simulink model "platoon_plus"  (R2020b)
settings: Solver=VariableStepAuto  StartTime=0.0  StopTime=120  RelTol=1e-3
values from neighbouring files (symbols this model uses):
  d_0 = 8    [platoon.m]
  Ka = 0.55    [platoon.m]
  Kd_err_pl = 0.401    [platoon.m]
  Kv = 0.5    [platoon.m]
  Kv_r_pl = 0.56    [platoon.m]
  t_h_tar = 1    [platoon.m]
  v_initial = [30 25 28 27]    [platoon.m]
  v_tar = 30    [platoon.m]
  x_initial = [150 100 50 0]    [platoon.m]
libraries: simulink x8
settings Model: Creator=alessandro  LastModifiedBy=gabriele

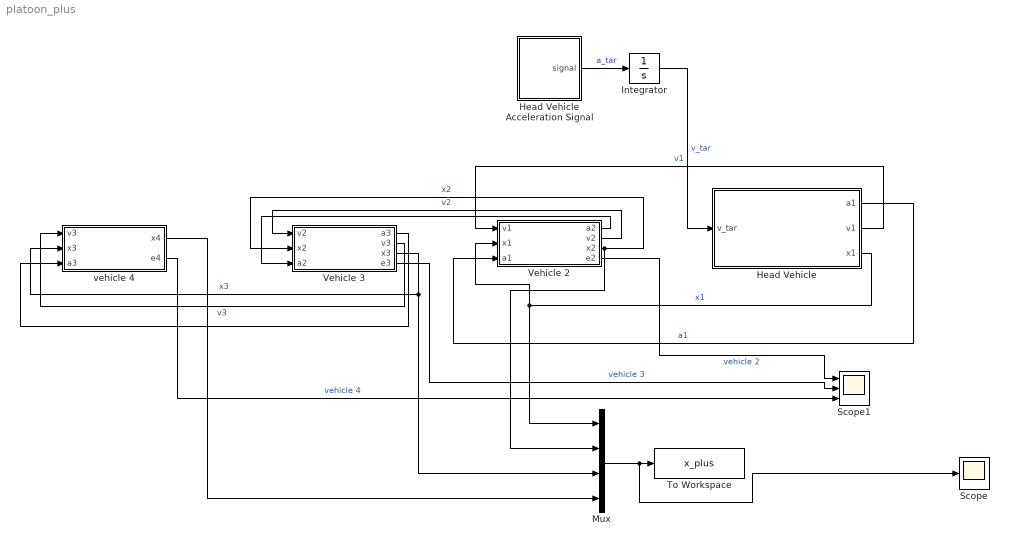
== system platoon_plus ==
  "Head Vehicle " : Subsystem
  Head Vehicle Acceleration Signal : Subsystem
  Integrator : Integrator  InitialCondition=v_initial(1)
  Mux : Mux
  Scope : Scope
  Scope1 : Scope  NumInputPorts=3
  To Workspace : ToWorkspace  VariableName=x_plus  SampleTime=-1
  Vehicle 2 : Subsystem
  Vehicle 3 : Subsystem
  vehicle 4 : Subsystem
  wires:
  Mux/1 -> Scope/1, To Workspace/1
  Vehicle 2/2(v2) -> Vehicle 3/1(v2)  "v2"
  Head Vehicle Acceleration Signal/1(signal) -> Integrator/1  "a_tar"
  vehicle 4/1(x4) -> Mux/4
  "Head Vehicle "/2(v1) -> Vehicle 2/1(v1)  "v1"
  Vehicle 3/2(v3) -> vehicle 4/1(v3)  "v3"
  Integrator/1 -> "Head Vehicle "/1(v_tar)  "v_tar"
  Vehicle 2/3(x2) -> Mux/2, Vehicle 3/2(x2)  "x2"
  "Head Vehicle "/3(x1) -> Mux/1, Vehicle 2/2(x1)  "x1"
  Vehicle 3/3(x3) -> Mux/3, vehicle 4/2(x3)  "x3"
  "Head Vehicle "/1(a1) -> Vehicle 2/3(a1)  "a1"
  Vehicle 2/1(a2) -> Vehicle 3/3(a2)
  Vehicle 3/1(a3) -> vehicle 4/3(a3)
  Vehicle 2/4(e2) -> Scope1/1  "vehicle 2"
  Vehicle 3/4(e3) -> Scope1/2  "vehicle 3"
  vehicle 4/2(e4) -> Scope1/3  "vehicle 4"

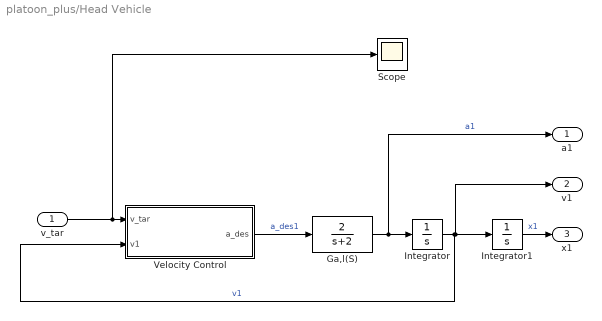
== system platoon_plus/Head Vehicle  ==
  v_tar : Inport
  Ga,l(S) : TransferFcn  Numerator=[2]  Denominator=[1 2]
  Integrator : Integrator  InitialCondition=v_initial(1)
  Integrator1 : Integrator  InitialCondition=x_initial(1)
  Scope : Scope
  Velocity Control : Subsystem
  a1 : Outport
  v1 : Outport  Port=2
  x1 : Outport  Port=3
  wires:
  Integrator/1 -> Velocity Control/2(v1), v1/1, Integrator1/1  "v1"
  Ga,l(S)/1 -> a1/1, Integrator/1  "a1"
  v_tar/1 -> Scope/1, Velocity Control/1(v_tar)
  Velocity Control/1(a_des) -> Ga,l(S)/1  "a_des1"
  Integrator1/1 -> x1/1  "x1"

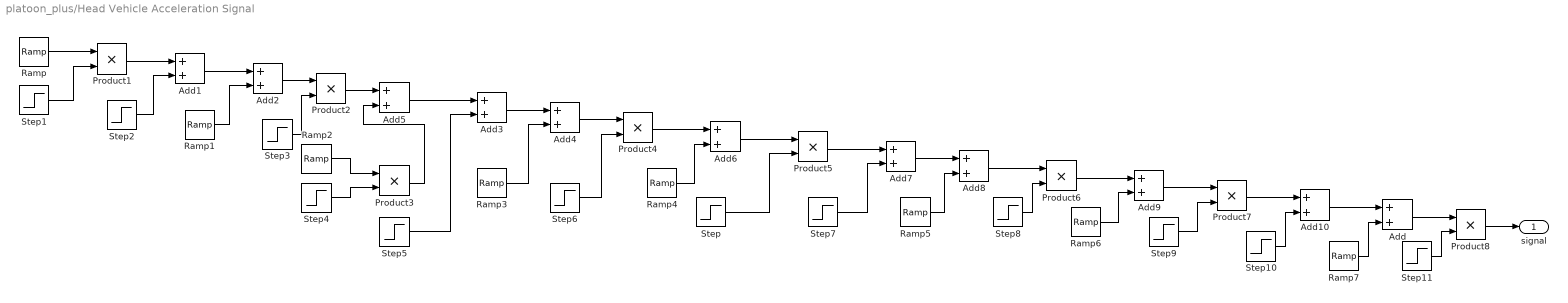
== system platoon_plus/Head Vehicle Acceleration Signal ==
  Add{,1..10} (11 alike) : Sum
  Product{1..8} (8 alike) : Product
  Ramp : simulink/Sources/Ramp  slope=-4  start=10  InitialOutput=0
  Ramp1 : simulink/Sources/Ramp  slope=4  start=13.5  InitialOutput=0
  Ramp2 : simulink/Sources/Ramp  slope=4  start=40  InitialOutput=0
  Ramp3 : simulink/Sources/Ramp  slope=-4  start=43.5  InitialOutput=0
  Ramp4 : simulink/Sources/Ramp  slope=-4  start=70  InitialOutput=0
  Ramp5 : simulink/Sources/Ramp  slope=4  start=73.5  InitialOutput=0
  Ramp6 : simulink/Sources/Ramp  slope=4  start=100  InitialOutput=0
  Ramp7 : simulink/Sources/Ramp  slope=-4  start=103.5  InitialOutput=0
  Step : Step  Time=70.5  Before=1  After=0  SampleTime=0
  Step1 : Step  Time=10.5  Before=1  After=0  SampleTime=0.1
  Step10 : Step  Time=100.5  After=2  SampleTime=0
  Step11 : Step  Time=104  Before=1  After=0  SampleTime=0
  Step2 : Step  Time=10.5  After=-2  SampleTime=0
  Step3 : Step  Time=14  Before=1  After=0  SampleTime=0
  Step4 : Step  Time=40.5  Before=1  After=0  SampleTime=0
  Step5 : Step  Time=40.5  After=2  SampleTime=0
  Step6 : Step  Time=44  Before=1  After=0  SampleTime=0
  Step7 : Step  Time=70.5  After=-2  SampleTime=0
  Step8 : Step  Time=74  Before=1  After=0  SampleTime=0
  Step9 : Step  Time=100.5  Before=1  After=0  SampleTime=0
  signal : Outport
  wires:
  Add1/1 -> Add2/1
  Step3/1 -> Product2/2
  Product3/1 -> Add5/2
  Step5/1 -> Add3/2
  Add2/1 -> Product2/1
  Step1/1 -> Product1/2
  Product2/1 -> Add5/1
  Step2/1 -> Add1/2
  Ramp2/1 -> Product3/1
  Product1/1 -> Add1/1
  Add4/1 -> Product4/1
  Ramp/1 -> Product1/1
  Add3/1 -> Add4/1
  Step6/1 -> Product4/2
  Ramp1/1 -> Add2/2
  Step4/1 -> Product3/2
  Add5/1 -> Add3/1
  Ramp3/1 -> Add4/2
  Product4/1 -> Add6/1
  Ramp4/1 -> Add6/2
  Add6/1 -> Product5/1
  Step/1 -> Product5/2
  Product5/1 -> Add7/1
  Step7/1 -> Add7/2
  Add7/1 -> Add8/1
  Ramp5/1 -> Add8/2
  Add8/1 -> Product6/1
  Step8/1 -> Product6/2
  Product6/1 -> Add9/1
  Ramp6/1 -> Add9/2
  Add9/1 -> Product7/1
  Step9/1 -> Product7/2
  Step10/1 -> Add10/2
  Product7/1 -> Add10/1
  Add10/1 -> Add/1
  Ramp7/1 -> Add/2
  Add/1 -> Product8/1
  Step11/1 -> Product8/2
  Product8/1 -> signal/1

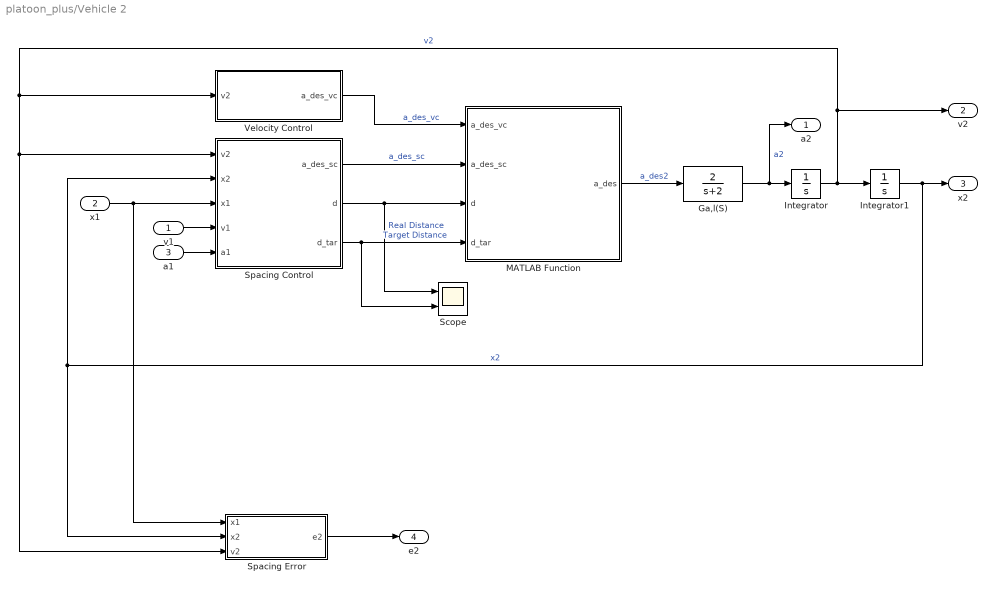
== system platoon_plus/Vehicle 2 ==
  v1 : Inport
  x1 : Inport  Port=2
  a1 : Inport  Port=3
  Ga,l(S) : TransferFcn  Numerator=[2]  Denominator=[1 2]
  Integrator : Integrator  InitialCondition=v_initial(2)
  Integrator1 : Integrator  InitialCondition=x_initial(2)
  MATLAB Function : MATLAB Function  TreatAsAtomicUnit=on
  Scope : Scope  NumInputPorts=2
  Spacing Control : Subsystem
  Spacing Error : Subsystem
  Velocity Control : Subsystem
  a2 : Outport
  v2 : Outport  Port=2
  x2 : Outport  Port=3
  e2 : Outport  Port=4
  wires:
  Spacing Control/1(a_des_sc) -> MATLAB Function/2(a_des_sc)  "a_des_sc"
  Velocity Control/1(a_des_vc) -> MATLAB Function/1(a_des_vc)  "a_des_vc"
  v1/1 -> Spacing Control/4(v1)
  x1/1 -> Spacing Control/3(x1), Spacing Error/1(x1)
  Spacing Control/2(d) -> Scope/1, MATLAB Function/3(d)  "Real Distance"
  MATLAB Function/1(a_des) -> Ga,l(S)/1  "a_des2"
  Integrator1/1 -> x2/1, Spacing Control/2(x2), Spacing Error/2(x2)  "x2"
  Spacing Control/3(d_tar) -> Scope/2, MATLAB Function/4(d_tar)  "Target Distance"
  Ga,l(S)/1 -> a2/1, Integrator/1  "a2"
  Integrator/1 -> Integrator1/1, v2/1, Velocity Control/1(v2), Spacing Control/1(v2), Spacing Error/3(v2)  "v2"
  Spacing Error/1(e2) -> e2/1
  a1/1 -> Spacing Control/5(a1)

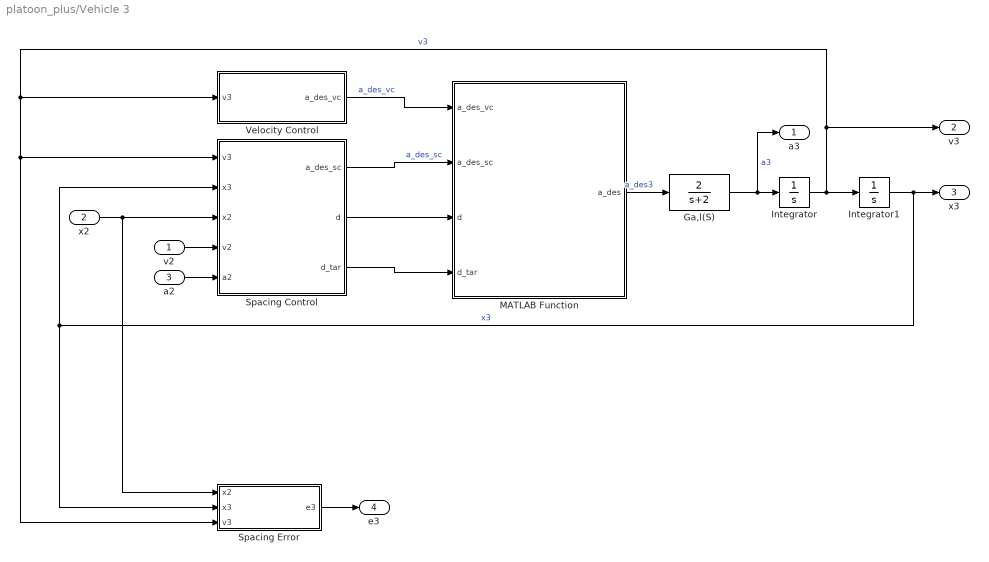
== system platoon_plus/Vehicle 3 ==
  v2 : Inport
  x2 : Inport  Port=2
  a2 : Inport  Port=3
  Ga,l(S) : TransferFcn  Numerator=[2]  Denominator=[1 2]
  Integrator : Integrator  InitialCondition=v_initial(3)
  Integrator1 : Integrator  InitialCondition=x_initial(3)
  MATLAB Function : MATLAB Function  TreatAsAtomicUnit=on
  Spacing Control : Subsystem
  Spacing Error : Subsystem
  Velocity Control : Subsystem
  a3 : Outport
  v3 : Outport  Port=2
  x3 : Outport  Port=3
  e3 : Outport  Port=4
  wires:
  Spacing Control/1(a_des_sc) -> MATLAB Function/2(a_des_sc)  "a_des_sc"
  Velocity Control/1(a_des_vc) -> MATLAB Function/1(a_des_vc)  "a_des_vc"
  v2/1 -> Spacing Control/4(v2)
  x2/1 -> Spacing Control/3(x2), Spacing Error/1(x2)
  Spacing Control/2(d) -> MATLAB Function/3(d)
  MATLAB Function/1(a_des) -> Ga,l(S)/1  "a_des3"
  Integrator1/1 -> x3/1, Spacing Control/2(x3), Spacing Error/2(x3)  "x3"
  Spacing Control/3(d_tar) -> MATLAB Function/4(d_tar)
  Ga,l(S)/1 -> a3/1, Integrator/1  "a3"
  Integrator/1 -> Integrator1/1, v3/1, Velocity Control/1(v3), Spacing Error/3(v3), Spacing Control/1(v3)  "v3"
  Spacing Error/1(e3) -> e3/1
  a2/1 -> Spacing Control/5(a2)

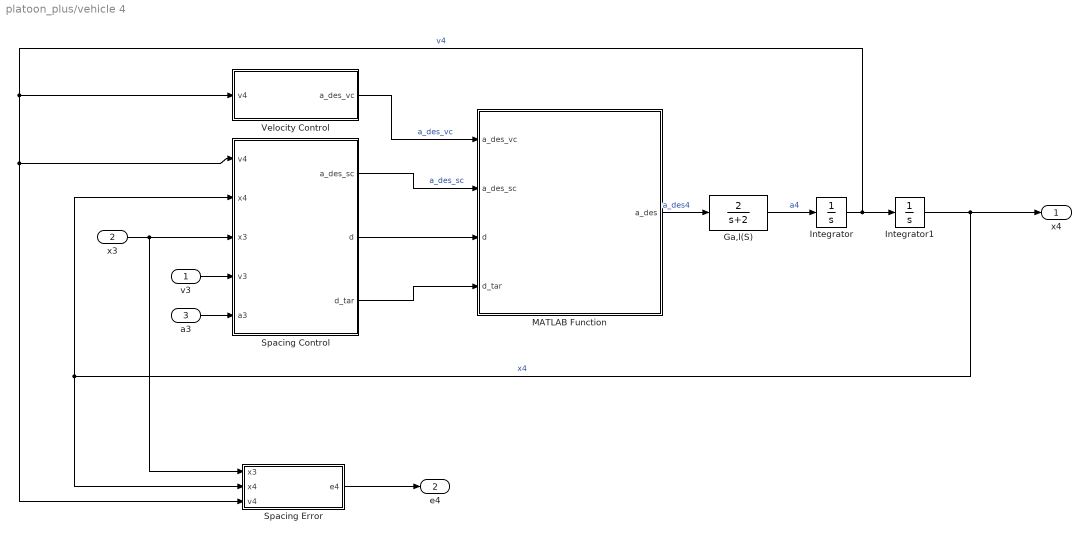
== system platoon_plus/vehicle 4 ==
  v3 : Inport
  x3 : Inport  Port=2
  a3 : Inport  Port=3
  Ga,l(S) : TransferFcn  Numerator=[2]  Denominator=[1 2]
  Integrator : Integrator  InitialCondition=v_initial(4)
  Integrator1 : Integrator  InitialCondition=x_initial(4)
  MATLAB Function : MATLAB Function  TreatAsAtomicUnit=on
  Spacing Control : Subsystem
  Spacing Error : Subsystem
  Velocity Control : Subsystem
  x4 : Outport
  e4 : Outport  Port=2
  wires:
  Spacing Control/1(a_des_sc) -> MATLAB Function/2(a_des_sc)  "a_des_sc"
  Velocity Control/1(a_des_vc) -> MATLAB Function/1(a_des_vc)  "a_des_vc"
  v3/1 -> Spacing Control/4(v3)
  x3/1 -> Spacing Error/1(x3), Spacing Control/3(x3)
  Spacing Control/2(d) -> MATLAB Function/3(d)
  MATLAB Function/1(a_des) -> Ga,l(S)/1  "a_des4"
  Integrator1/1 -> Spacing Control/2(x4), Spacing Error/2(x4), x4/1  "x4"
  Spacing Control/3(d_tar) -> MATLAB Function/4(d_tar)
  Ga,l(S)/1 -> Integrator/1  "a4"
  Integrator/1 -> Integrator1/1, Velocity Control/1(v4), Spacing Error/3(v4), Spacing Control/1(v4)  "v4"
  Spacing Error/1(e4) -> e4/1
  a3/1 -> Spacing Control/5(a3)

== system platoon_plus/Head Vehicle /Velocity Control ==
  v_tar : Inport
  v1 : Inport  Port=2
  Gain : Gain  Gain=Kv
  Subtract : Sum  Inputs=+-
  a_des : Outport
  wires:
  v1/1 -> Subtract/2
  v_tar/1 -> Subtract/1
  Subtract/1 -> Gain/1  "e_v"
  Gain/1 -> a_des/1  "a_des"

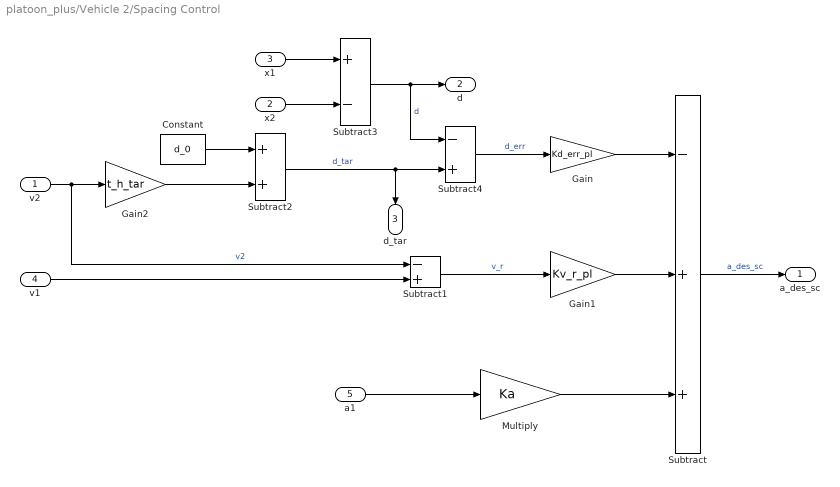
== system platoon_plus/Vehicle 2/Spacing Control ==
  v2 : Inport
  x2 : Inport  Port=2
  x1 : Inport  Port=3
  v1 : Inport  Port=4
  a1 : Inport  Port=5
  Constant : Constant  Value=d_0
  Gain : Gain  Gain=Kd_err_pl
  Gain1 : Gain  Gain=Kv_r_pl
  Gain2 : Gain  Gain=t_h_tar
  Multiply : Gain  Gain=Ka
  Subtract : Sum  Inputs=-++
  Subtract1 : Sum  Inputs=-+
  Subtract2 : Sum
  Subtract3 : Sum  Inputs=+-
  Subtract4 : Sum  Inputs=-+
  a_des_sc : Outport
  d : Outport  Port=2
  d_tar : Outport  Port=3
  wires:
  Gain/1 -> Subtract/1
  Gain1/1 -> Subtract/2
  Subtract/1 -> a_des_sc/1  "a_des_sc"
  v2/1 -> Subtract1/1, Gain2/1  "v2"
  Subtract1/1 -> Gain1/1  "v_r"
  Gain2/1 -> Subtract2/2
  v1/1 -> Subtract1/2
  x1/1 -> Subtract3/1
  x2/1 -> Subtract3/2
  Subtract2/1 -> Subtract4/2, d_tar/1  "d_tar"
  Subtract3/1 -> Subtract4/1, d/1  "d"
  Subtract4/1 -> Gain/1  "d_err"
  Constant/1 -> Subtract2/1
  a1/1 -> Multiply/1
  Multiply/1 -> Subtract/3

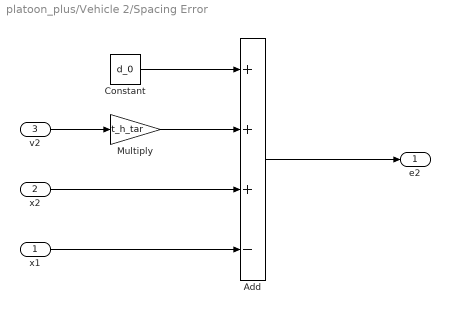
== system platoon_plus/Vehicle 2/Spacing Error ==
  x1 : Inport
  x2 : Inport  Port=2
  v2 : Inport  Port=3
  Add : Sum  Inputs=+++-
  Constant : Constant  Value=d_0
  Multiply : Gain  Gain=t_h_tar
  e2 : Outport
  wires:
  Constant/1 -> Add/1
  Multiply/1 -> Add/2
  v2/1 -> Multiply/1
  x2/1 -> Add/3
  x1/1 -> Add/4
  Add/1 -> e2/1

== system platoon_plus/Vehicle 2/Velocity Control ==
  v2 : Inport
  Constant : Constant  Value=v_tar
  Gain : Gain  Gain=Kv
  Subtract : Sum  Inputs=+-
  a_des_vc : Outport
  wires:
  v2/1 -> Subtract/2
  Constant/1 -> Subtract/1
  Subtract/1 -> Gain/1  "e_v"
  Gain/1 -> a_des_vc/1  "a_des_vc"

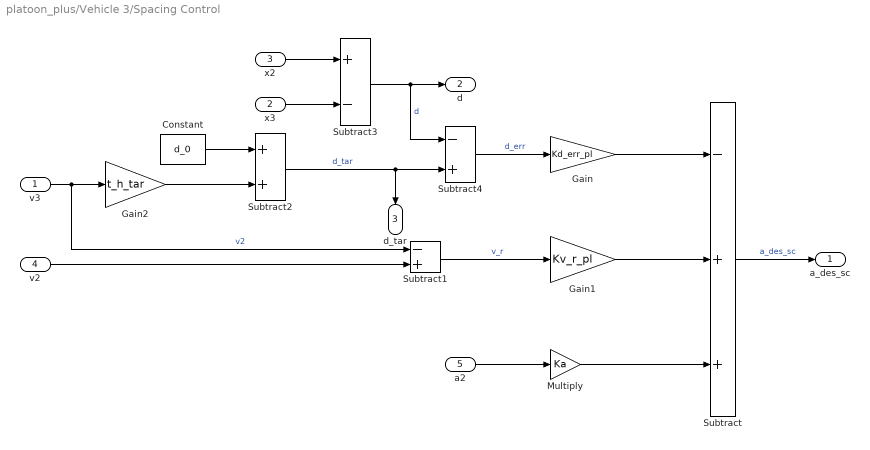
== system platoon_plus/Vehicle 3/Spacing Control ==
  v3 : Inport
  x3 : Inport  Port=2
  x2 : Inport  Port=3
  v2 : Inport  Port=4
  a2 : Inport  Port=5
  Constant : Constant  Value=d_0
  Gain : Gain  Gain=Kd_err_pl
  Gain1 : Gain  Gain=Kv_r_pl
  Gain2 : Gain  Gain=t_h_tar
  Multiply : Gain  Gain=Ka
  Subtract : Sum  Inputs=-++
  Subtract1 : Sum  Inputs=-+
  Subtract2 : Sum
  Subtract3 : Sum  Inputs=+-
  Subtract4 : Sum  Inputs=-+
  a_des_sc : Outport
  d : Outport  Port=2
  d_tar : Outport  Port=3
  wires:
  Gain/1 -> Subtract/1
  Gain1/1 -> Subtract/2
  Subtract/1 -> a_des_sc/1  "a_des_sc"
  v3/1 -> Subtract1/1, Gain2/1  "v2"
  Subtract1/1 -> Gain1/1  "v_r"
  Gain2/1 -> Subtract2/2
  v2/1 -> Subtract1/2
  x2/1 -> Subtract3/1
  x3/1 -> Subtract3/2
  Subtract2/1 -> Subtract4/2, d_tar/1  "d_tar"
  Subtract3/1 -> Subtract4/1, d/1  "d"
  Subtract4/1 -> Gain/1  "d_err"
  Constant/1 -> Subtract2/1
  a2/1 -> Multiply/1
  Multiply/1 -> Subtract/3

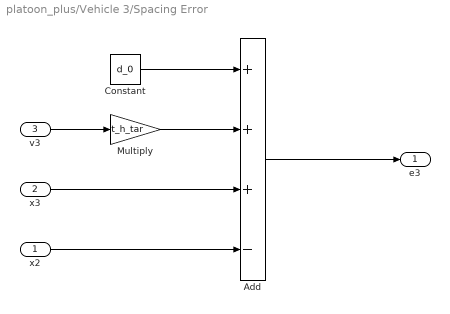
== system platoon_plus/Vehicle 3/Spacing Error ==
  x2 : Inport
  x3 : Inport  Port=2
  v3 : Inport  Port=3
  Add : Sum  Inputs=+++-
  Constant : Constant  Value=d_0
  Multiply : Gain  Gain=t_h_tar
  e3 : Outport
  wires:
  Constant/1 -> Add/1
  Multiply/1 -> Add/2
  v3/1 -> Multiply/1
  x3/1 -> Add/3
  x2/1 -> Add/4
  Add/1 -> e3/1

== system platoon_plus/Vehicle 3/Velocity Control ==
  v3 : Inport
  Constant : Constant  Value=v_tar
  Gain : Gain  Gain=Kv
  Subtract : Sum  Inputs=+-
  a_des_vc : Outport
  wires:
  v3/1 -> Subtract/2
  Constant/1 -> Subtract/1
  Subtract/1 -> Gain/1  "e_v"
  Gain/1 -> a_des_vc/1  "a_des_vc"

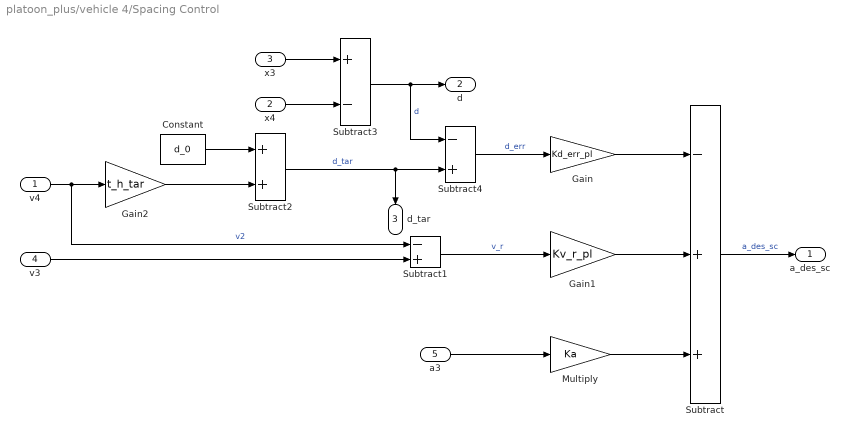
== system platoon_plus/vehicle 4/Spacing Control ==
  v4 : Inport
  x4 : Inport  Port=2
  x3 : Inport  Port=3
  v3 : Inport  Port=4
  a3 : Inport  Port=5
  Constant : Constant  Value=d_0
  Gain : Gain  Gain=Kd_err_pl
  Gain1 : Gain  Gain=Kv_r_pl
  Gain2 : Gain  Gain=t_h_tar
  Multiply : Gain  Gain=Ka
  Subtract : Sum  Inputs=-++
  Subtract1 : Sum  Inputs=-+
  Subtract2 : Sum
  Subtract3 : Sum  Inputs=+-
  Subtract4 : Sum  Inputs=-+
  a_des_sc : Outport
  d : Outport  Port=2
  d_tar : Outport  Port=3
  wires:
  Gain/1 -> Subtract/1
  Gain1/1 -> Subtract/2
  Subtract/1 -> a_des_sc/1  "a_des_sc"
  v4/1 -> Subtract1/1, Gain2/1  "v2"
  Subtract1/1 -> Gain1/1  "v_r"
  Gain2/1 -> Subtract2/2
  v3/1 -> Subtract1/2
  x3/1 -> Subtract3/1
  x4/1 -> Subtract3/2
  Subtract2/1 -> Subtract4/2, d_tar/1  "d_tar"
  Subtract3/1 -> Subtract4/1, d/1  "d"
  Subtract4/1 -> Gain/1  "d_err"
  Constant/1 -> Subtract2/1
  a3/1 -> Multiply/1
  Multiply/1 -> Subtract/3

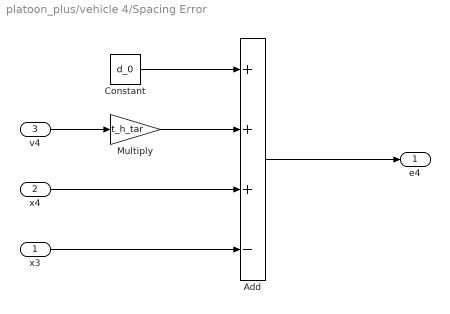
== system platoon_plus/vehicle 4/Spacing Error ==
  x3 : Inport
  x4 : Inport  Port=2
  v4 : Inport  Port=3
  Add : Sum  Inputs=+++-
  Constant : Constant  Value=d_0
  Multiply : Gain  Gain=t_h_tar
  e4 : Outport
  wires:
  Constant/1 -> Add/1
  Multiply/1 -> Add/2
  v4/1 -> Multiply/1
  x4/1 -> Add/3
  x3/1 -> Add/4
  Add/1 -> e4/1

== system platoon_plus/vehicle 4/Velocity Control ==
  v4 : Inport
  Constant : Constant  Value=v_tar
  Gain : Gain  Gain=Kv
  Subtract : Sum  Inputs=+-
  a_des_vc : Outport
  wires:
  v4/1 -> Subtract/2
  Constant/1 -> Subtract/1
  Subtract/1 -> Gain/1  "e_v"
  Gain/1 -> a_des_vc/1  "a_des_vc"

== matlab function platoon_plus/Vehicle 2/MATLAB Function ==
  data: a_des_vc input; a_des output; a_des_sc input; d input; d_tar input
function a_des = switching_logic(a_des_vc, a_des_sc, d, d_tar)

if d > d_tar
    a_des = min([a_des_vc a_des_sc]);
else
    a_des = a_des_sc;
end

if a_des > 5 
    a_des = 5;
end

if a_des < -3
    a_des = -3;
end


end

== matlab function platoon_plus/Vehicle 3/MATLAB Function ==
  data: a_des_vc input; a_des output; a_des_sc input; d input; d_tar input
function a_des = switching_logic(a_des_vc, a_des_sc, d, d_tar)

if d > d_tar
    a_des = min([a_des_vc a_des_sc]);
else
    a_des = a_des_sc;
end

if a_des > 5 
    a_des = 5;
end

if a_des < -3
    a_des = -3;
end


end

== matlab function platoon_plus/vehicle 4/MATLAB Function ==
  data: a_des_vc input; a_des output; a_des_sc input; d input; d_tar input
function a_des = switching_logic(a_des_vc, a_des_sc, d, d_tar)

if d > d_tar
    a_des = min([a_des_vc a_des_sc]);
else
    a_des = a_des_sc;
end

if a_des > 5 
    a_des = 5;
end

if a_des < -3
    a_des = -3;
end


end
